simulink model "Q2_UAV"  (R2022a)
settings: Solver=VariableStepAuto  StartTime=0.0  StopTime=10  RelTol=1e-3
settings Model: Creator=Eshmith  LastModifiedBy=Eshmith

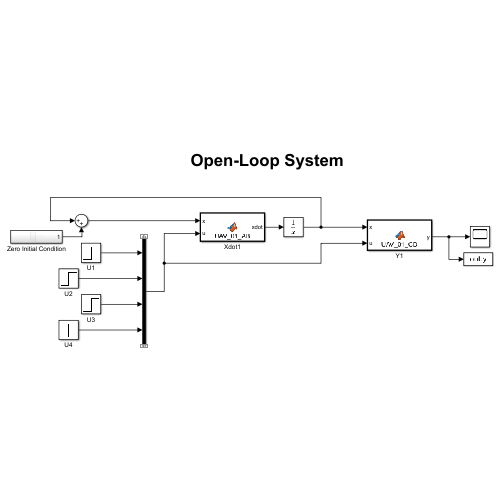
[thumbnail: Simulink's stored preview of the top-level diagram]
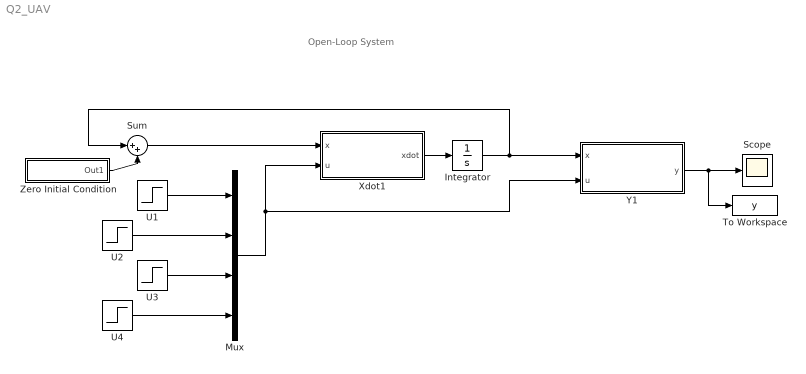
== system Q2_UAV ==
  note: Open-Loop System
  Integrator : Integrator
  Mux : Mux
  Scope : Scope
  Sum : Sum  Inputs=|++
  To Workspace : ToWorkspace  VariableName=y  SaveFormat=Timeseries  SampleTime=-1
  U1 : Step  Time=0  SampleTime=0
  U2 : Step  Time=0  After=0  SampleTime=0
  U3 : Step  After=0  SampleTime=0
  U4 : Step  After=0  SampleTime=0
  Xdot1 : MATLAB Function  TreatAsAtomicUnit=on
  Y1 : MATLAB Function  TreatAsAtomicUnit=on
  Zero Initial Condition : Subsystem
  wires:
  Xdot1/1(xdot) -> Integrator/1
  U1/1 -> Mux/1
  Mux/1 -> Y1/2(u), Xdot1/2(u)
  Integrator/1 -> Y1/1(x), Sum/1
  Y1/1(y) -> To Workspace/1, Scope/1
  Sum/1 -> Xdot1/1(x)
  Zero Initial Condition/1(Out1) -> Sum/2
  U2/1 -> Mux/2
  U3/1 -> Mux/3
  U4/1 -> Mux/4

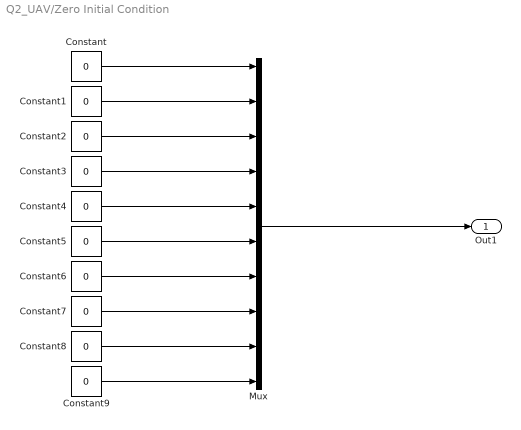
== system Q2_UAV/Zero Initial Condition ==
  Constant{,1..9} (10 alike) : Constant  Value=0
  Mux : Mux  Inputs=10
  Out1 : Outport
  wires:
  Mux/1 -> Out1/1
  Constant5/1 -> Mux/6
  Constant7/1 -> Mux/8
  Constant2/1 -> Mux/3
  Constant9/1 -> Mux/10
  Constant3/1 -> Mux/4
  Constant8/1 -> Mux/9
  Constant1/1 -> Mux/2
  Constant/1 -> Mux/1
  Constant4/1 -> Mux/5
  Constant6/1 -> Mux/7

== matlab function Q2_UAV/Xdot1 ==
  data: x input; u input; xdot output
function xdot = UAV_01_AB(x, u)


A_long =[[-0.5944,0.8008,-9.791,-0.8747,5.077*10^(-5)];
         [-0.744,-7.56,-0.5294,15.72,-0.000939];
         [0,0,0,1,0];
         [1.041,-7.406,0,-15.81,-7.284*10^(-18)];
         [-0.05399,0.9985,-17,0,0]];

B_long = [[0.4669,0];
          [-2.703,0];
          [0,0];
          [-133.7,0];
          [0,0]];

C_long = [[0.9985,0.05399,0,0,0];
          [-003176,0.05874,0,0,0];
          [0,0,0,1,0];
          [0,0,1,0,0];
          [0,0,0,0,-1]];



A_lat = [[-0.8726,0.8789,-16.82,9.791,0];
         [-2.823,-16.09,3.367,0,0];
         [0.702,0.514,-2.775,0,0];
         [0,1,0.05406,-4.088*10^(-24),0];
         [0,0,1.001,-7.573*10^(-23),0]];

B_lat = [[0,5.302];
         [-156.5,-5.008];
         [11.5,-82.04];
         [0,0];
         [0,0]];

C_lat = [[0.05882,0,0,0,0];
         [0,1,0,0,0];
         [0,0,1,0,0];
         [0,0,0,1,0];
         [0,0,0,0,1]];


A = [A_long , zeros(size(A_long,1), size(A_lat,2)); zeros(size(A_lat,1), size(A_long,2)), A_lat];
B = [B_long , zeros(size(B_long,1), size(B_lat,2)); zeros(size(B_lat,1), size(B_long,2)), B_lat];
C = [C_long , zeros(size(C_long,1), size(C_lat,2)); zeros(size(C_lat,1), size(C_long,2)), C_lat];
D = zeros(size(C,1),size(B,2));

K = ones(4, 10);

xdot = A*x + B*u;

end

== matlab function Q2_UAV/Y1 ==
  data: x input; u input; y output
function y = UAV_01_CD(x, u)


A_long =[[-0.5944,0.8008,-9.791,-0.8747,5.077*10^(-5)];
         [-0.744,-7.56,-0.5294,15.72,-0.000939];
         [0,0,0,1,0];
         [1.041,-7.406,0,-15.81,-7.284*10^(-18)];
         [-0.05399,0.9985,-17,0,0]];

B_long = [[0.4669,0];
          [-2.703,0];
          [0,0];
          [-133.7,0];
          [0,0]];

C_long = [[0.9985,0.05399,0,0,0];
          [-003176,0.05874,0,0,0];
          [0,0,0,1,0];
          [0,0,1,0,0];
          [0,0,0,0,-1]];



A_lat = [[-0.8726,0.8789,-16.82,9.791,0];
         [-2.823,-16.09,3.367,0,0];
         [0.702,0.514,-2.775,0,0];
         [0,1,0.05406,-4.088*10^(-24),0];
         [0,0,1.001,-7.573*10^(-23),0]];

B_lat = [[0,5.302];
         [-156.5,-5.008];
         [11.5,-82.04];
         [0,0];
         [0,0]];

C_lat = [[0.05882,0,0,0,0];
         [0,1,0,0,0];
         [0,0,1,0,0];
         [0,0,0,1,0];
         [0,0,0,0,1]];


A = [A_long , zeros(size(A_long,1), size(A_lat,2)); zeros(size(A_lat,1), size(A_long,2)), A_lat];
B = [B_long , zeros(size(B_long,1), size(B_lat,2)); zeros(size(B_lat,1), size(B_long,2)), B_lat];
C = [C_long , zeros(size(C_long,1), size(C_lat,2)); zeros(size(C_lat,1), size(C_long,2)), C_lat];
D = zeros(size(C,1),size(B,2));

K = ones(4, 10);

y = C*x + D*u;

end
